simulink model "ParentApp"  (R2023b)
settings: Solver=FixedStepAuto  StartTime=0.0  StopTime=inf  RelTol=1e-3
undefined symbols (not defined in the file): Button, lat, Latitude, long, Longitude, ParentsApp, Reset
libraries: androidcommunicationlib x7, androiduilib x5, androidaudiovideolib x3
settings Model: Creator=raj54  LastModifiedBy=Dell
settings OptimizationCC: EnhancedBackFolding=on  PassReuseOutputArgsThreshold=0  MaxStackSize=64  OptimizeBlockOrder=speed  DifferentSizesBufferReuse=on  OptimizationCustomize=off
settings DebuggingCC: ParameterTunabilityLossMsg=error
settings HardwareCC: ProdBitPerPointer=32  ProdBitPerSizeT=32  ProdBitPerPtrDiffT=32  ProdLargestAtomicInteger=Long  ProdLargestAtomicFloat=Double  ProdWordSize=32  ProdHWDeviceType=ARM Compatible->ARM Cortex  UseEmbeddedCoderFeatures=off  UseSimulinkCoderFeatures=off
settings ModelReferenceCC: EnableRefExpFcnMdlSchedulingChecks=on
settings SFSimCC: MATLABDynamicMemAlloc=off
settings RTWCC: Description=Embedded Coder  SystemTargetFile=ert.tlc  HardwareBoard=Android Device  TLCOptions="-aInlineSetEventsForThisBaseRateFcn=TLC_FALSE -aSuppressMultiTaskScheduler=TLC_FALSE  -aRateBasedStepFcn=0"  TemplateMakefile=ert_default_tmf  RTWVerbose=off  Toolchain=Android SDK/NDK Tools
settings CodeAppCC: ForceParamTrailComments=on  OperatorAnnotations=on
settings ERTTargetCC: ERTCustomFileBanners=off  SupportContinuousTime=on  SupportNonInlinedSFcns=on  RemoveResetFunc=off  ModelStepFunctionPrototypeControlCompliant=off

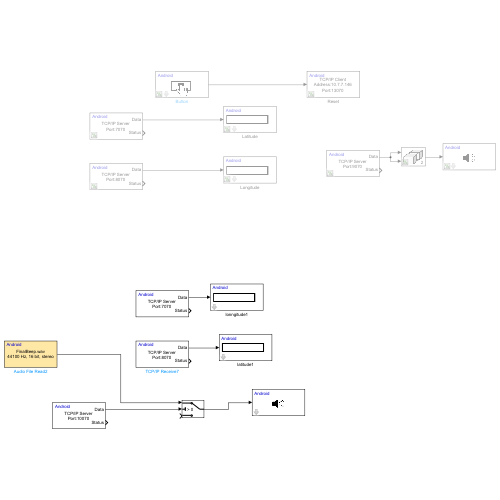
[thumbnail: Simulink's stored preview of the top-level diagram]
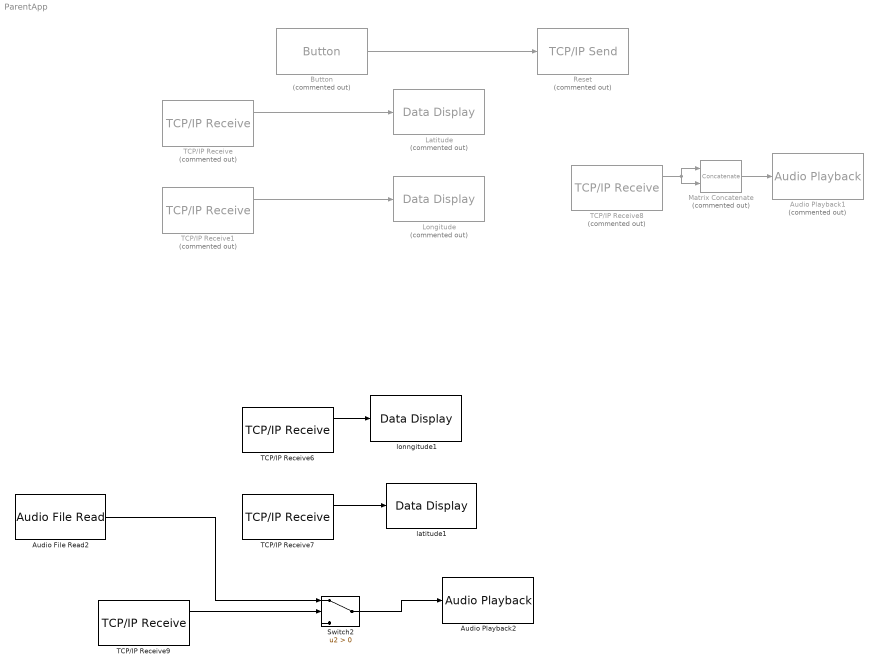
== system ParentApp ==
  Audio File Read2 : androidaudiovideolib/Audio File Read  FileName=C:\Users\Dell\Downloads\FinalBeep.wav  FrameSize=4410
  Audio Playback1 : androidaudiovideolib/Audio Playback  Commented=on  SampleFreq=44100  AudioSamplingFreq=44100  SampleTime=0.1  DeviceStr=0  QueueDuration=0  BlockPlatform=Android
  Audio Playback2 : androidaudiovideolib/Audio Playback  SampleFreq=44100  AudioSamplingFreq=44100  SampleTime=0.1  DeviceStr=0  QueueDuration=0  BlockPlatform=Android
  Button : androiduilib/Button  Commented=on  ButtonState=Not pressed  ButtonId=ParentsApp/Button  State=off  SampleTime=0.1  BlockPlatform=Android
  Latitude : androiduilib/Data Display  Commented=on  DataDisplayId=ParentsApp/Latitude  Format=Float  Precision=6  SimulateUsing=Code generation  blockPlatform=Android
  Longitude : androiduilib/Data Display  Commented=on  DataDisplayId=ParentsApp/Longitude  Format=Float  Precision=6  SimulateUsing=Code generation  blockPlatform=Android
  Matrix Concatenate : Concatenate  Commented=on  Mode=Multidimensional array  ConcatenateDimension=2
  Reset : androidcommunicationlib/TCP//IP Send  Commented=on  TCPSendId=ParentsApp/Reset  Mode_=Client  LocalServerPort_=25000  RemoteAddr_=10.7.7.146  RemoteServerPort_=13070  ClientPortBindingSelection_=off  ClientPortToBind_=35000  BlockingMode_=off  BlockTimeout_=0.1
  Switch2 : Switch  Criteria=u2 > Threshold  SaturateOnIntegerOverflow=off  InputSameDT=off
  TCP/IP Receive : androidcommunicationlib/TCP//IP Receive  Commented=on  TCPReceiveId=ParentsApp/TCP//IP_Receive  Mode_=Server  LocalServerPort_=7070  RemoteAddr_=127.0.0.1  RemoteServerPort_=25000  DataType_=uint8  DataSize_=1  SampleTime_=4  ClientPortBindingSelection_=off  ClientPortToBind_=35000  BlockingMode_=on  BlockTimeout_=4.1
  TCP/IP Receive1 : androidcommunicationlib/TCP//IP Receive  Commented=on  TCPReceiveId=ParentsApp/TCP//IP_Receive1  Mode_=Server  LocalServerPort_=8070  RemoteAddr_=127.0.0.1  RemoteServerPort_=25000  DataType_=uint8  DataSize_=1  SampleTime_=4  ClientPortBindingSelection_=off  ClientPortToBind_=35000  BlockingMode_=on  BlockTimeout_=4.1
  TCP/IP Receive6 : androidcommunicationlib/TCP//IP Receive  TCPReceiveId=ParentsApp/TCP//IP_Receive6  Mode_=Server  LocalServerPort_=7070  RemoteAddr_=127.0.0.1  RemoteServerPort_=25000  DataType_=uint8  DataSize_=1  SampleTime_=4  ClientPortBindingSelection_=off  ClientPortToBind_=35000  BlockingMode_=on  BlockTimeout_=4.1
  TCP/IP Receive7 : androidcommunicationlib/TCP//IP Receive  TCPReceiveId=ParentsApp/TCP//IP_Receive7  Mode_=Server  LocalServerPort_=8070  RemoteAddr_=127.0.0.1  RemoteServerPort_=25000  DataType_=uint8  DataSize_=1  SampleTime_=4  ClientPortBindingSelection_=off  ClientPortToBind_=35000  BlockingMode_=on  BlockTimeout_=4.1
  TCP/IP Receive8 : androidcommunicationlib/TCP//IP Receive  Commented=on  TCPReceiveId=ParentsApp/TCP//IP_Receive8  Mode_=Server  LocalServerPort_=9070  RemoteAddr_=127.0.0.1  RemoteServerPort_=25000  DataType_=int16  DataSize_=1  SampleTime_=4  ClientPortBindingSelection_=off  ClientPortToBind_=35000  BlockingMode_=on  BlockTimeout_=4.1
  TCP/IP Receive9 : androidcommunicationlib/TCP//IP Receive  TCPReceiveId=ParentsApp/TCP//IP_Receive9  Mode_=Server  LocalServerPort_=10070  RemoteAddr_=127.0.0.1  RemoteServerPort_=25000  DataType_=uint8  DataSize_=1  SampleTime_=4  ClientPortBindingSelection_=off  ClientPortToBind_=35000  BlockingMode_=on  BlockTimeout_=4.1
  latitude1 : androiduilib/Data Display  DataDisplayId=ParentsApp/lat  Format=Float  Precision=6  SimulateUsing=Code generation  blockPlatform=Android
  lonngitude1 : androiduilib/Data Display  DataDisplayId=ParentsApp/long  Format=Float  Precision=6  SimulateUsing=Code generation  blockPlatform=Android
  wires:
  TCP/IP Receive/1 -> Latitude/1
  TCP/IP Receive1/1 -> Longitude/1
  Button/1 -> Reset/1
  TCP/IP Receive7/1 -> latitude1/1
  TCP/IP Receive6/1 -> lonngitude1/1
  Matrix Concatenate/1 -> Audio Playback1/1
  TCP/IP Receive8/1 -> Matrix Concatenate/1, Matrix Concatenate/2
  Switch2/1 -> Audio Playback2/1
  TCP/IP Receive9/1 -> Switch2/2
  Audio File Read2/1 -> Switch2/1
